simulink model "PMSM"  (R2015b)
settings: Solver=ode4  StartTime=0.0  StopTime=2  FixedStep=5e-06  RelTol=1e-5  AbsTol=1e-3
undefined symbols (not defined in the file or in its folder): DiscIntNeverNeededParam
libraries: dspmtrx3 x11, aerolibutil x7, simulink x4, simulink_extras x4, commnoisgen2 x2, dspinverses x1
(part 1 of 2)
settings Model: Creator=Сергей  LastModifiedBy=acsl
settings SolverCC: ZeroCrossAlgorithm=Adaptive
settings DataIOCC: FinalStateName=pmsm_fstate  InitialState=pmsm_fstate  LimitDataPoints=off  SaveFinalState=on  SaveCompleteFinalSimState=on  SaveFormat=Array  SignalLoggingSaveFormat=ModelDataLogs  SaveOutput=off  SignalLogging=off  DSMLogging=off  SaveTime=off  ReturnWorkspaceOutputs=on  ReturnWorkspaceOutputsName=output
settings OptimizationCC: ExpressionDepthLimit=2147483647
settings DebuggingCC: SaveWithDisabledLinksMsg=none  SaveWithParameterizedLinksMsg=none  UnderspecifiedInitializationDetection=Classic  MergeDetectMultiDrivingBlocksExec=none  SolverPrmCheckMsg=warning  Int32ToFloatConvMsg=none  FcnCallInpInsideContextMsg=EnableAllAsWarning  UnconnectedInputMsg=none  UnconnectedOutputMsg=none  UnconnectedLineMsg=none  BusObjectLabelMismatch=none  RootOutportRequireBusObject=none  ModelReferenceDataLoggingMessage=none  StateNameClashWarn=warning  SFUnusedDataAndEventsDiag=none  SFUnexpectedBacktrackingDiag=none  SFInvalidInputDataAccessInChartInitDiag=none  SFNoUnconditionalDefaultTransitionDiag=none  SFTransitionOutsideNaturalParentDiag=none  SFUnconditionalTransitionShadowingDiag=none  SFUndirectedBroadcastEventsDiag=none  SFTransitionActionBeforeConditionDiag=none
settings HardwareCC: ProdBitPerPointer=32  ProdLargestAtomicFloat=None  ProdIntDivRoundTo=Undefined  ProdEndianess=Unspecified  ProdWordSize=32  ProdHWDeviceType=32-bit Generic
settings GRTTargetCC: GeneratePreprocessorConditionals=Disable all  CombineOutputUpdateFcns=off  GRTInterface=on
settings ConfigComp: CovModelRefEnable=Off

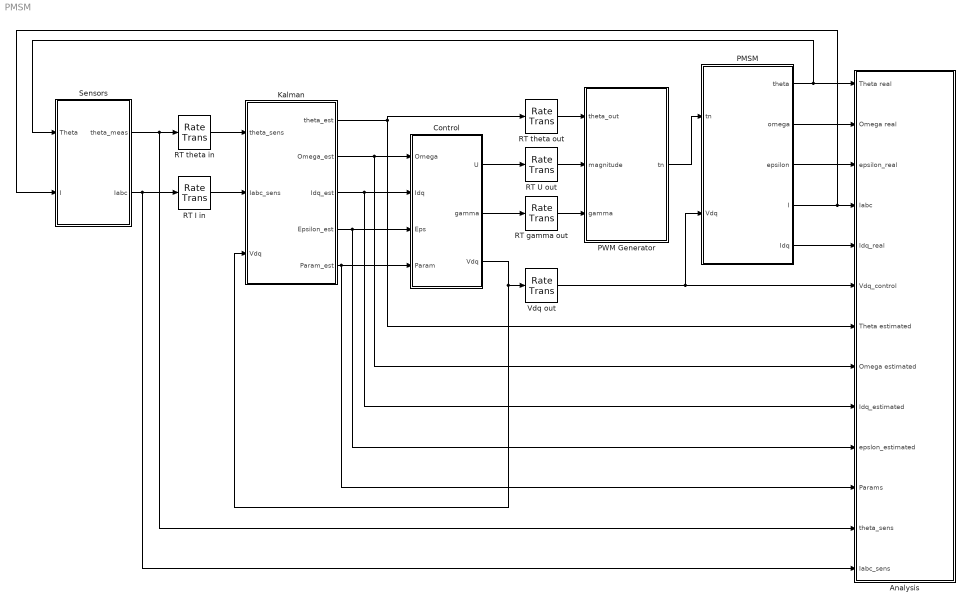
== system PMSM ==
  Analysis : Subsystem  mask{sampleTime=5e-05}
      mask prompts: sampleTime "Sample time"
  Control : Subsystem  TreatAsAtomicUnit=on  SystemSampleTime=5e-05  mask{CT=Torque control, DV=100, DT=0.06, Vs=12, R=0.4, L=0.0001, J=0.008, Kt=0.011, Kf=0.0001, Tr=2e-4, Tr_omega=1e-2, Tr_trq=3e-4, Imax=20, Wmax=110, controlST=5e-05}
      mask prompts: CT "Control type"; DV "Desired angular velocity, rev/min"; DT "Desired torque, Nm"; Vs "Nominal voltage (assumed in a model), V"; R "Coil resistance (assumed in a model), Ohm"; L "Coil inductance (assumed in a model), H"; J "Rotor inertia (assumed in a model), kg*m^2"; Kt "Torque constant (assumed in a model), N*m/A"; Kf "Viscous Friction constant (assumed in a model), N*m*s"; Tr "Rise time (velocity)"; Tr_omega "Rise time (omega)"; Tr_trq "Rise time (torque)"; Imax "I constraint"; Wmax "W constraint"; controlST "Control Sample Time"
      settings: MinAlgLoopOccurrences=on
      mask TypeOptions CT: Velocity control | Torque control
      mask Callback CT:
      | sys_name=gcs;
      | b = get_param(strcat(sys_name,'/Control'),'MaskValues');
      | a = get_param(strcat(sys_name,'/Control'),'MaskVisibilities');
      | if strcmp(b(1), 'Torque control')
      |     a{2}='off';
      |     a{3}='on';
      | end
      | if strcmp(b(1), 'Velocity control')
      |     a{2}='on';
      |     a{3}='off';
      | end
      | set_param(strcat(sys_name,'/Control'),'MaskVisibilities',a);
  Kalman : Subsystem  TreatAsAtomicUnit=on  SystemSampleTime=5e-05  mask{aaaaaa=off, Vs_r=12, Vs=12, R_r=0.3, R=0.4, L_r=0.0001, L=0.0001, J_r=0.008, J=0.008, Kt_r=0.011, Kt=0.011, Kf_r=0.001509, Kf=0.0001, Kc_r=0.010142, Kc=0.01, source=Mask, I_0=[0 0 0], I_0_r=[1 2 -3], theta0=0, theta0_r=0, w0=0, w0_r=0, eps0=0, eps0_r=0, kalmanST=5e-05}
      mask prompts: aaaaaa "Assume model parameters equal to real"; Vs_r "Nominal voltage, V"; Vs "Nominal voltage (assumed in a model), V"; R_r "Coil resistance, Ohm"; R "Coil resistance (assumed in a model), Ohm"; L_r "Coil inductance, H"; L "Coil inductance (assumed in a model), H"; J_r "Rotor inertia, kg*m^2"; J "Rotor inertia (assumed in a model), kg*m^2"; Kt_r "Torque constant, N*m/A"; Kt "Torque constant (assumed in a model), N*m/A"; Kf_r "Viscous Friction constant, N*m*s"; Kf "Viscous Friction constant (assumed in a model), N*m*s"; Kc_r "Coulomb Friction constant, N*m"; Kc "Coulomb Friction constant (assumed in a model), N*m"; source "Angle and Current initial conditions source"; I_0 "Initial currents ABC, A (assumed in a model), A"; I_0_r "Initial currents ABC, A"; theta0 "Initial angle (assumed in a model), deg"; theta0_r "Initial angle, deg"; w0 "Initial angular velocity (assumed in a model), rev/min"; w0_r "Initial angular velocity, rev/min"; eps0 "Initial angular acceleration (assumed in a model), rad/sec^2"; eps0_r "Initial angular acceleration, rad/sec^2"; kalmanST "Kalman Sample Tine"
      mask init:
      | sys_name=gcs;
      | ap = get_param(strcat(sys_name,'/PMSM'),'MaskPrompts');
      | bp = get_param(strcat(sys_name,'/Kalman'),'MaskPrompts');
      | cp = get_param(strcat(sys_name,'/Control'),'MaskPrompts');
      | a = get_param(strcat(sys_name,'/PMSM'),'MaskValues');
      | b = get_param(strcat(sys_name,'/Kalman'),'MaskValues');
      | c = get_param(strcat(sys_name,'/Control'),'MaskValues');
      | 
      | for i=1:length(ap)
      |     for j=1:length(bp)
      |         if strcmp(ap(i),bp(j))
      |             a(i)=b(j);
      |         end
      |     end
      | end
      | 
      | for i=1:length(bp)
      |     for j=1:length(cp)
      |         if strcmp(bp(i),cp(j))
      |             c(j)=b(i);
      |         end
      |     end
      | end
      | 
      | set_param(strcat(sys_name,'/PMSM'),'MaskValues',a);
      | set_param(strcat(sys_name,'/Control'),'MaskValues',c);
      settings: MinAlgLoopOccurrences=on
      mask Callback aaaaaa:
      | sys_name=gcs;
      | b = get_param(strcat(sys_name,'/Kalman'),'MaskValues');
      | 
      | if strcmp(b(1),'on')
      |     for i=3:2:19
      |         b(i)=b(i-1);
      |     end
      | end
      | 
      | set_param(strcat(sys_name,'/Kalman'),'MaskValues',b);
      mask TypeOptions source: Mask | Sensors
      mask Callback source:
      | sys_name=gcs;
      | b = get_param(strcat(sys_name,'/Kalman'),'MaskValues');
      | a = get_param(strcat(sys_name,'/Kalman'),'MaskEnables');
      | if strcmp(b(16), 'Mask')
      |     a{17}='on';
      |     a{19}='on';
      | end
      | if strcmp(b(16), 'Sensors')
      |     a{17}='off';
      |     a{19}='off';
      | end
      | set_param(strcat(sys_name,'/Kalman'),'MaskEnables',a);
  PMSM : Subsystem  mask{Vs=12, R=0.3, L=0.0001, J=0.008, Kt=0.011, Kf=0.001509, Kc=0.010142, s=0.9e-3, ws=1e-3, I_0=[1 2 -3], theta0=0, w0=0, eps0=0, delta_phin=[0 0 0]}
      mask prompts: Vs "Nominal voltage, V"; R "Coil resistance, Ohm"; L "Coil inductance, H"; J "Rotor inertia, kg*m^2"; Kt "Torque constant, N*m/A"; Kf "Viscous Friction constant, N*m*s"; Kc "Coulomb Friction constant, N*m"; s "Stribeck coeffitient, N*m"; ws "Stribeck velosity, 1/s"; I_0 "Initial currents ABC, A"; theta0 "Initial angle, deg"; w0 "Initial angular velocity, rev/min"; eps0 "Initial angular acceleration, rad/sec^2"; delta_phin "Error in phases angles, deg"
  PWM Generator : Subsystem  mask{f=40000, Vs=12}
      mask prompts: f "PWM fequency, Hz"; Vs "Nominal voltage, V"
  RT I in : RateTransition  OutPortSampleTime=5e-05
  RT U out : RateTransition  OutPortSampleTime=5e-06
  RT gamma out : RateTransition  OutPortSampleTime=5e-06
  RT theta in : RateTransition  OutPortSampleTime=5e-05
  RT theta out : RateTransition  OutPortSampleTime=5e-06
  Sensors : Subsystem  mask{I_n=[0.05 0.05 0.05], I_b=[0 0 0], D_I=0.05, h_n=[0.6 0.6 0.6]*2, h_b=[0 0 0], h_A=[3800 3800 3800], h_o=[2000 2000 2000], rrr=off, hb=[0 0 0], hA=[3800 3800 3800], ho=[2000 2000 2000], h1l=[1000 3000], h2l=[1000 3000], h3l=[1000 3000]}
      mask prompts: I_n "Coil currents fluctation error [I1 I2 I3] (3 sigma), A"; I_b "Coil currents bias [I1 I2 I3], A"; D_I "Coil currents ADC digit size, A"; h_n "Hall sensors fluctation error [H1 H2 H3] (3 sigma), ADC digits"; h_b "Hall sensors  bias [H1 H2 H3], deg"; h_A "Hall sesors ADC digits amplitude [H1 H2 H3],  ADC digits"; h_o "Hall sensors ADC digit cetral line offset [H1 H2 H3], ADC digits"; rrr "Assume etimated parameters equal to real"; hb "Hall sensors  bias [H1 H2 H3], deg"; hA "Hall sesors ADC digits amplitude [H1 H2 H3],  ADC digits"; ho "Hall sensors ADC digit cetral line offset [H1 H2 H3], ADC digits"; h1l "Hall sensor 1 trust limit"; h2l "Hall sensor 2 trust limit"; h3l "Hall sensor 3 trust limit"
      mask init:
      | ap = get_param('PMSM/Sensors','MaskPrompts');
      | a = get_param('PMSM/Sensors','MaskValues');
      | 
      | if strcmp(a(8), 'on')
      |     
      | for i=1:length(ap)
      |     for j=i:length(ap)
      |         if strcmp(ap(i),ap(j))
      |             a(j)=a(i);
      |         end
      |     end
      | end
      | 
      | end
      | 
      | set_param('PMSM/Sensors','MaskValues',a);
      mask Callback rrr:
      | sys_name=gcs;
      | ap = get_param(strcat(sys_name,'/Sensors'),'MaskPrompts');
      | a = get_param(strcat(sys_name,'/Sensors'),'MaskValues');
      | 
      | if strcmp(a(8), 'on')
      | 
      | for i=1:length(ap)
      |     for j=i:length(ap)
      |         if strcmp(ap(i),ap(j))
      |             a(j)=a(i);
      |         end
      |     end
      | end
      | 
      | end
      | 
      | set_param(strcat(sys_name,'/Sensors'),'MaskValues',a);
  Vdq out : RateTransition  OutPortSampleTime=5e-06
  wires:
  PMSM/2(omega) -> Analysis/2(Omega real)
  PMSM/3(epsilon) -> Analysis/3(epsilon_real)
  Kalman/2(Omega_est) -> Analysis/8(Omega estimated), Control/1(Omega)
  Kalman/1(theta_est) -> Analysis/7(Theta estimated), RT theta out/1
  Kalman/3(Idq_est) -> Analysis/9(Idq_estimated), Control/2(Idq)
  PMSM/5(Idq) -> Analysis/5(Idq_real)
  Kalman/4(Epsilon_est) -> Analysis/10(epslon_estimated), Control/3(Eps)
  Control/3(Vdq) -> Kalman/3(Vdq), Vdq out/1
  PWM Generator/1(tn) -> PMSM/1(tn)
  Control/2(gamma) -> RT gamma out/1
  Control/1(U) -> RT U out/1
  RT U out/1 -> PWM Generator/2(magnitude)
  RT gamma out/1 -> PWM Generator/3(gamma)
  Vdq out/1 -> PMSM/2(Vdq), Analysis/6(Vdq_control)
  PMSM/1(theta) -> Sensors/1(Theta), Analysis/1(Theta real)
  PMSM/4(I) -> Sensors/2(I), Analysis/4(Iabc)
  Sensors/1(theta_meas) -> RT theta in/1, Analysis/12(theta_sens)
  Sensors/2(Iabc) -> RT I in/1, Analysis/13(Iabc_sens)
  RT theta in/1 -> Kalman/1(theta_sens)
  RT I in/1 -> Kalman/2(Iabc_sens)
  RT theta out/1 -> PWM Generator/1(theta_out)
  Kalman/5(Param_est) -> Analysis/11(Params), Control/4(Param)

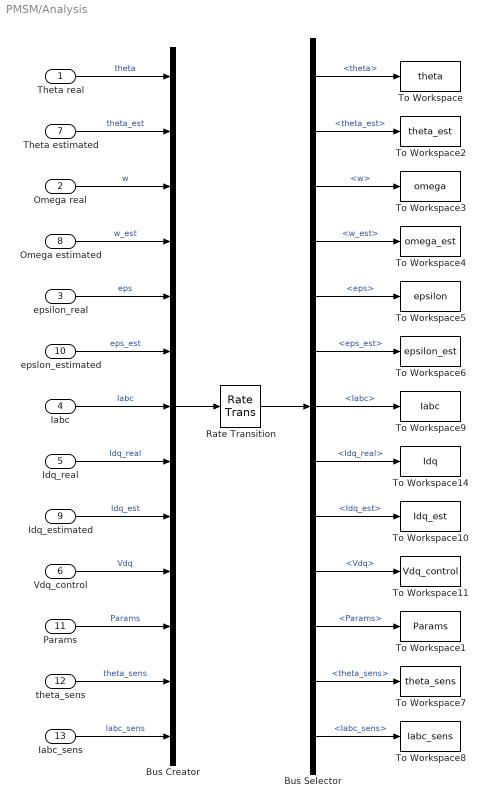
== system PMSM/Analysis ==
  Theta real : Inport
  Omega real : Inport  Port=2
  epsilon_real : Inport  Port=3
  Iabc : Inport  Port=4
  Idq_real : Inport  Port=5
  Vdq_control : Inport  Port=6
  Theta estimated : Inport  Port=7
  Omega estimated : Inport  Port=8
  Idq_estimated : Inport  Port=9
  epslon_estimated : Inport  Port=10
  Params : Inport  Port=11
  theta_sens : Inport  Port=12
  Iabc_sens : Inport  Port=13
  Bus Creator : BusCreator  Inputs=13
  Bus Selector : BusSelector  OutputSignals=theta,theta_est,w,w_est,eps,eps_est,Iabc,Idq_real,Idq_est,Vdq,Params,theta_sens,Iabc_sens
  Rate Transition : RateTransition  Deterministic=off  OutPortSampleTime=sampleTime
  To Workspace : ToWorkspace  VariableName=theta  SaveFormat=Timeseries  SampleTime=sampleTime
  To Workspace1 : ToWorkspace  VariableName=Params  SaveFormat=Timeseries  SampleTime=sampleTime
  To Workspace10 : ToWorkspace  VariableName=Idq_est  SaveFormat=Timeseries  SampleTime=sampleTime
  To Workspace11 : ToWorkspace  VariableName=Vdq_control  SaveFormat=Timeseries  SampleTime=sampleTime
  To Workspace14 : ToWorkspace  VariableName=Idq  SaveFormat=Timeseries  SampleTime=sampleTime
  To Workspace2 : ToWorkspace  VariableName=theta_est  SaveFormat=Timeseries  SampleTime=sampleTime
  To Workspace3 : ToWorkspace  VariableName=omega  SaveFormat=Timeseries  SampleTime=sampleTime
  To Workspace4 : ToWorkspace  VariableName=omega_est  SaveFormat=Timeseries  SampleTime=sampleTime
  To Workspace5 : ToWorkspace  VariableName=epsilon  SaveFormat=Timeseries  SampleTime=sampleTime
  To Workspace6 : ToWorkspace  VariableName=epsilon_est  SaveFormat=Timeseries  SampleTime=sampleTime
  To Workspace7 : ToWorkspace  VariableName=theta_sens  SaveFormat=Timeseries  SampleTime=sampleTime
  To Workspace8 : ToWorkspace  VariableName=Iabc_sens  SaveFormat=Timeseries  SampleTime=sampleTime
  To Workspace9 : ToWorkspace  VariableName=Iabc  SaveFormat=Timeseries  SampleTime=sampleTime
  wires:
  Theta estimated/1 -> Bus Creator/2  "theta_est"
  Theta real/1 -> Bus Creator/1  "theta"
  epsilon_real/1 -> Bus Creator/5  "eps"
  Iabc/1 -> Bus Creator/7  "Iabc"
  Bus Creator/1 -> Rate Transition/1
  Rate Transition/1 -> Bus Selector/1
  Bus Selector/1 -> To Workspace/1  "<theta>"
  Omega real/1 -> Bus Creator/3  "w"
  epslon_estimated/1 -> Bus Creator/6  "eps_est"
  Idq_estimated/1 -> Bus Creator/9  "Idq_est"
  Vdq_control/1 -> Bus Creator/10  "Vdq"
  Bus Selector/3 -> To Workspace3/1  "<w>"
  Bus Selector/4 -> To Workspace4/1  "<w_est>"
  Bus Selector/5 -> To Workspace5/1  "<eps>"
  Bus Selector/6 -> To Workspace6/1  "<eps_est>"
  Bus Selector/7 -> To Workspace9/1  "<Iabc>"
  Bus Selector/9 -> To Workspace10/1  "<Idq_est>"
  Bus Selector/10 -> To Workspace11/1  "<Vdq>"
  Omega estimated/1 -> Bus Creator/4  "w_est"
  Idq_real/1 -> Bus Creator/8  "Idq_real"
  Bus Selector/8 -> To Workspace14/1  "<Idq_real>"
  Bus Selector/2 -> To Workspace2/1  "<theta_est>"
  Params/1 -> Bus Creator/11  "Params"
  Bus Selector/11 -> To Workspace1/1  "<Params>"
  theta_sens/1 -> Bus Creator/12  "theta_sens"
  Iabc_sens/1 -> Bus Creator/13  "Iabc_sens"
  Bus Selector/12 -> To Workspace7/1  "<theta_sens>"
  Bus Selector/13 -> To Workspace8/1  "<Iabc_sens>"

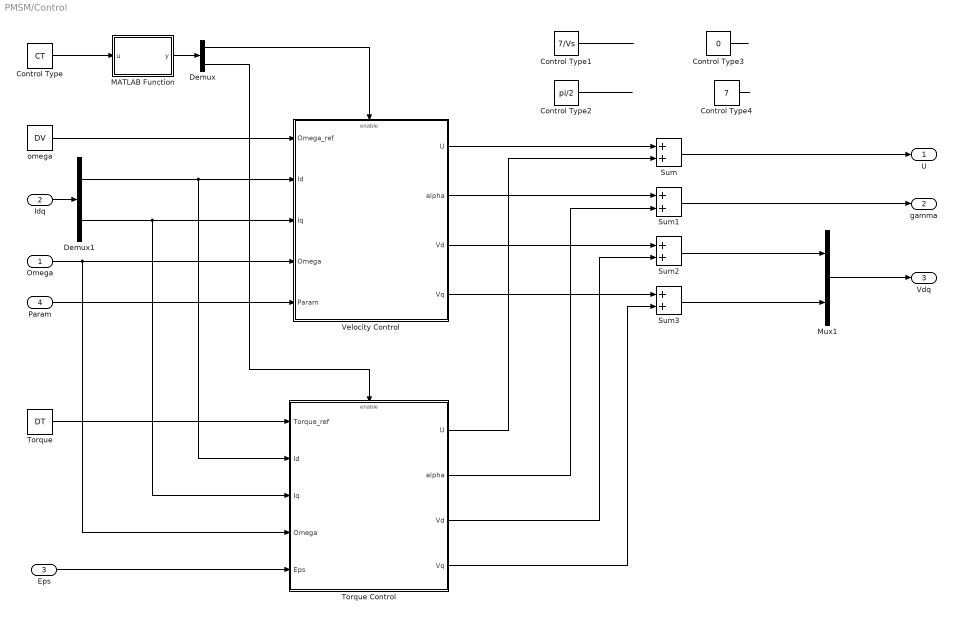
== system PMSM/Control ==
  Omega : Inport
  Idq : Inport  Port=2
  Eps : Inport  Port=3
  Param : Inport  Port=4
  Control Type : Constant  Value=CT
  Control Type1 : Constant  Value=7/Vs
  Control Type2 : Constant  Value=pi/2
  Control Type3 : Constant  Value=0
  Control Type4 : Constant  Value=7
  Demux : Demux  Outputs=2
  Demux1 : Demux  Outputs=2
  MATLAB Function : MATLAB Function  TreatAsAtomicUnit=on
  Mux1 : Mux  Inputs=2
  Sum{,1..3} (4 alike) : Sum
  Torque : Constant  Value=DT
  Torque Control : Subsystem
  Velocity Control : Subsystem
  omega : Constant  Value=DV
  U : Outport
  gamma : Outport  Port=2
  Vdq : Outport  Port=3
  wires:
  omega/1 -> Velocity Control/1(Omega_ref)
  Omega/1 -> Torque Control/4(Omega), Velocity Control/4(Omega)
  Velocity Control/1(U) -> Sum/1
  Velocity Control/2(alpha) -> Sum1/1
  Velocity Control/3(Vd) -> Sum2/1
  Velocity Control/4(Vq) -> Sum3/1
  Control Type/1 -> MATLAB Function/1(u)
  Torque/1 -> Torque Control/1(Torque_ref)
  MATLAB Function/1(y) -> Demux/1
  Demux/1 -> Velocity Control/Enable
  Torque Control/1(U) -> Sum/2
  Torque Control/2(alpha) -> Sum1/2
  Torque Control/3(Vd) -> Sum2/2
  Torque Control/4(Vq) -> Sum3/2
  Idq/1 -> Demux1/1
  Demux1/1 -> Torque Control/2(Id), Velocity Control/2(Id)
  Demux1/2 -> Torque Control/3(Iq), Velocity Control/3(Iq)
  Sum/1 -> U/1
  Sum1/1 -> gamma/1
  Sum2/1 -> Mux1/1
  Sum3/1 -> Mux1/2
  Eps/1 -> Torque Control/5(Eps)
  Control Type3/1 -> ?
  Control Type4/1 -> ?
  Demux/2 -> Torque Control/Enable
  Control Type1/1 -> ?
  Control Type2/1 -> ?
  Mux1/1 -> Vdq/1
  Param/1 -> Velocity Control/5(Param)

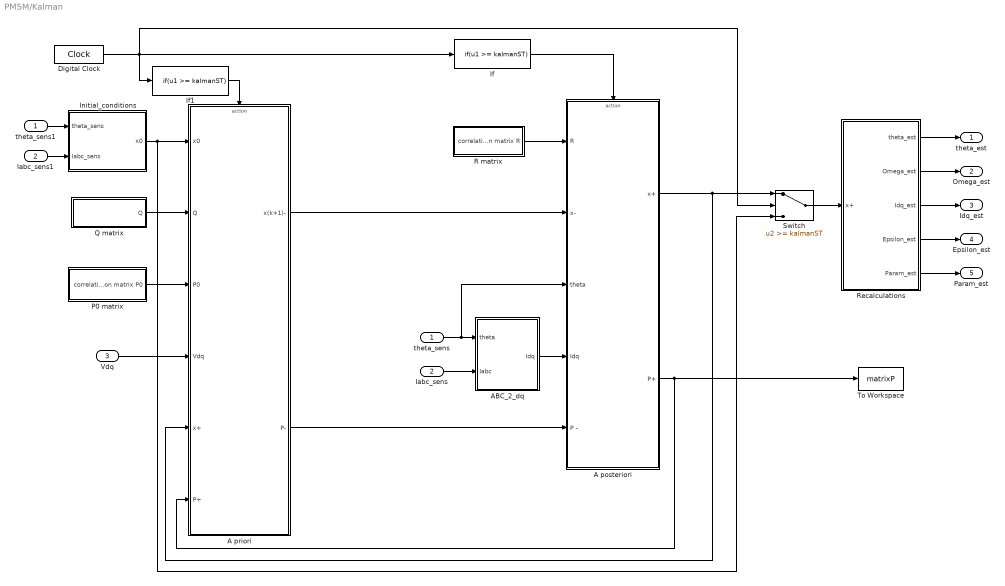
== system PMSM/Kalman ==
  theta_sens : Inport
  Iabc_sens : Inport  Port=2
  Vdq : Inport  Port=3
  A posteriori : Subsystem
  A priori : Subsystem
  ABC_2_dq : Subsystem
  Digital Clock : DigitalClock  SampleTime=kalmanST
  Iabc_sens1 : InportShadow  Port=2
  If : If  IfExpression=u1 >= kalmanST  ShowElse=off
  If1 : If  IfExpression=u1 >= kalmanST  ShowElse=off
  Initial_conditions : Subsystem
  P0 matrix : Subsystem
  Q matrix : Subsystem
  R matrix : Subsystem
  "Recalculations " : Subsystem
  Switch : Switch  Threshold=kalmanST
  To Workspace : ToWorkspace  VariableName=matrixP  SaveFormat=Timeseries  SampleTime=-1
  theta_sens1 : InportShadow
  theta_est : Outport
  Omega_est : Outport  Port=2
  Idq_est : Outport  Port=3
  Epsilon_est : Outport  Port=4
  Param_est : Outport  Port=5
  wires:
  A posteriori/1(x+) -> A priori/5(x+), Switch/1
  P0 matrix/1(correlation matrix P0) -> A priori/3(P0)
  A priori/1(x(k+1)-) -> A posteriori/2(x-)
  A posteriori/2(P+) -> To Workspace/1, A priori/6(P+)
  Q matrix/1(Q) -> A priori/2(Q)
  R matrix/1(correlation matrix R) -> A posteriori/1(R)
  A priori/2(P-) -> A posteriori/5(P -)
  theta_sens/1 -> A posteriori/3(theta), ABC_2_dq/1(theta)
  If/1 -> A posteriori/Action
  Vdq/1 -> A priori/4(Vdq)
  Digital Clock/1 -> Switch/2, If/1, If1/1
  If1/1 -> A priori/Action
  ABC_2_dq/1(Idq) -> A posteriori/4(Idq)
  Iabc_sens/1 -> ABC_2_dq/2(Iabc)
  "Recalculations "/4(Epsilon_est) -> Epsilon_est/1
  "Recalculations "/5(Param_est) -> Param_est/1
  "Recalculations "/3(Idq_est) -> Idq_est/1
  "Recalculations "/2(Omega_est) -> Omega_est/1
  "Recalculations "/1(theta_est) -> theta_est/1
  theta_sens1/1 -> Initial_conditions/1(theta_sens)
  Iabc_sens1/1 -> Initial_conditions/2(Iabc_sens)
  Switch/1 -> "Recalculations "/1(x+)
  Initial_conditions/1(x0) -> Switch/3, A priori/1(x0)

== system PMSM/PMSM ==
  tn : Inport
  Vdq : Inport  Port=2
  ABC_2_dq : Subsystem
  Degrees to Radians : simulink_extras/Transformations/Degrees to Radians
  Dot Product1 : DotProduct  InputSameDT=on  OutDataTypeStr=Inherit: Inherit via internal rule
  Kt : Gain  Gain=Kt
  Kt1 : Gain  Gain=-1
  Product : Product
  Rotor : Subsystem
  Stator : Subsystem
  Sum : Sum  Inputs=+++
  Trigonometric Function : Trigonometry
  dq_2_ABC : Subsystem
  phin : Constant  Value=[0 -2*pi/3 2*pi/3]
  phin1 : Constant  Value=delta_phin
  theta : Outport
  omega : Outport  Port=2
  epsilon : Outport  Port=3
  I : Outport  Port=4
  Idq : Outport  Port=5
  wires:
  Kt/1 -> Kt1/1, Product/1
  Rotor/3(omega) -> omega/1, Product/2
  Product/1 -> Stator/1(En)
  Trigonometric Function/1 -> Kt/1
  Sum/1 -> Trigonometric Function/1
  phin/1 -> Sum/2
  Dot Product1/1 -> Rotor/1(Te)
  Rotor/1(epsilon) -> epsilon/1
  Kt1/1 -> Dot Product1/1
  Rotor/2(theta) -> theta/1, ABC_2_dq/1(theta), dq_2_ABC/1(theta), Sum/3
  ABC_2_dq/1(Idq) -> Idq/1
  Stator/1(I) -> ABC_2_dq/2(Iabc), I/1, Dot Product1/2
  phin1/1 -> Degrees to Radians/1
  Degrees to Radians/1 -> Sum/1
  tn/1 -> Stator/2(tn)
  Vdq/1 -> dq_2_ABC/2(Vdq)
  dq_2_ABC/1(Vabc) -> Stator/3(Vabc)

== system PMSM/PWM Generator ==
  theta_out : Inport
  magnitude : Inport  Port=2
  gamma : Inport  Port=3
  Abs1 : Abs
  Constant1 : Constant  Value=0.5
  Constant2 : Constant  Value=pi/6
  ModFunction : Subsystem
  Product : Product
  Relational Operator1 : RelationalOperator  Operator=<=  OutDataTypeStr=boolean
  Sign : Signum
  Signal Generator1 : SignalGenerator  WaveForm=sawtooth  Frequency=f
  Sum1 : Sum  Inputs=|++
  Sum2 : Sum  Inputs=-+|
  Sum3 : Sum  Inputs=-+|
  Sum4 : Sum  Inputs=-+-
  phin : Constant  Value=[0 2*pi/3 4*pi/3]
  tn : Outport
  wires:
  gamma/1 -> Sum1/1
  phin/1 -> Sum4/1
  Sum2/1 -> Sign/1
  Constant1/1 -> Sum3/1, Sum2/1
  Signal Generator1/1 -> Abs1/1
  Constant2/1 -> Sum4/3
  ModFunction/1(Out1) -> Product/2
  Sum4/1 -> ModFunction/1(In1)
  Relational Operator1/1 -> Sum2/2
  Abs1/1 -> Sum3/2
  Sum3/1 -> Relational Operator1/1
  Product/1 -> Relational Operator1/2
  theta_out/1 -> Sum1/2
  magnitude/1 -> Product/1
  Sum1/1 -> Sum4/2
  Sign/1 -> tn/1

== system PMSM/Sensors ==
  Theta : Inport
  I : Inport  Port=2
  2Pi counter : Subsystem
  Demux : Demux  Outputs=3
  Gaussian Noise Generator : commnoisgen2/Gaussian Noise Generator  m=0  d=(I_n/3).^2  s=0  Ts=5e-06  frameBased=off  sampPerFrame=1  orient=off  outDataType=double
  Hall Sensor Coder : Subsystem
  Hall sensor decoder : Subsystem
  Mux : Mux  Inputs=3
  Quantizer : Quantizer  QuantizationInterval=D_I
  Sum1 : Sum  Inputs=+++
  bias currents : Constant  Value=I_b
  theta_meas : Outport
  Iabc : Outport  Port=2
  wires:
  Sum1/1 -> Quantizer/1
  Gaussian Noise Generator/1 -> Sum1/2
  Hall Sensor Coder/1(h) -> Hall sensor decoder/1(h)
  bias currents/1 -> Sum1/3
  Hall sensor decoder/1(theta_meas) -> 2Pi counter/1(Theta)
  Quantizer/1 -> Demux/1
  Demux/1 -> Mux/1
  Demux/3 -> Mux/3
  Demux/2 -> Mux/2
  I/1 -> Sum1/1
  Theta/1 -> Hall Sensor Coder/1(theta)
  2Pi counter/1(Theta_out) -> theta_meas/1
  Mux/1 -> Iabc/1

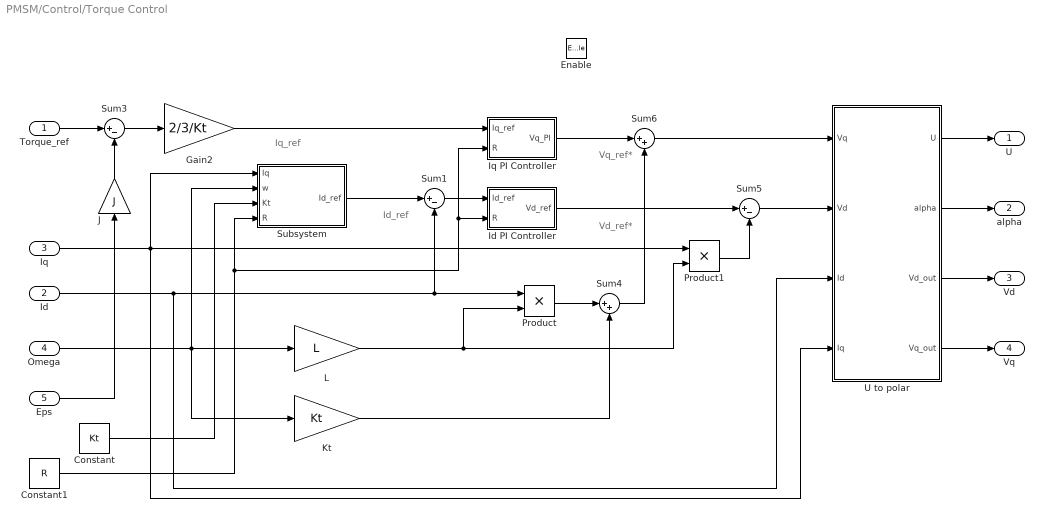
== system PMSM/Control/Torque Control ==
  note: Id_ref
  note: Iq_ref
  note: Vq_ref*
  note: Vd_ref*
  Torque_ref : Inport
  Id : Inport  Port=2
  Iq : Inport  Port=3
  Omega : Inport  Port=4
  Eps : Inport  Port=5
  Enable : EnablePort
  Constant : Constant  Value=Kt
  Constant1 : Constant  Value=R
  Gain2 : Gain  Gain=2/3/Kt
  Id PI Controller : Subsystem  mask{P=L/(Tr_trq*log(9)), I=R/(Tr_trq*log(9)), InitialConditionForIntegrator=0}
      mask prompts: P "Proportional Gain"; I "Integral Gain"; InitialConditionForIntegrator "Initial Condition For Integrator"
  Iq PI Controller : Subsystem  mask{P=L/(Tr_trq*log(9)), I=R/(Tr_trq*log(9)), InitialConditionForIntegrator=0}
      mask prompts: P "Proportional Gain"; I "Integral Gain"; InitialConditionForIntegrator "Initial Condition For Integrator"
  J : Gain  Gain=J
  Kt : Gain  Gain=Kt
  L : Gain  Gain=L
  Product : Product  RndMeth=Zero
  Product1 : Product  RndMeth=Zero
  Subsystem : Subsystem
  Sum1 : Sum  Inputs=|+-
  Sum3 : Sum  Inputs=|+-
  Sum4 : Sum  Inputs=|++
  Sum5 : Sum  Inputs=|+-
  Sum6 : Sum  Inputs=|++
  U to polar : Subsystem
  U : Outport
  alpha : Outport  Port=2
  Vd : Outport  Port=3
  Vq : Outport  Port=4
  wires:
  Sum6/1 -> U to polar/1(Vq)
  Sum3/1 -> Gain2/1
  U to polar/4(Vq_out) -> Vq/1
  U to polar/3(Vd_out) -> Vd/1
  U to polar/2(alpha) -> alpha/1
  U to polar/1(U) -> U/1
  Sum5/1 -> U to polar/2(Vd)
  Kt/1 -> Sum4/2
  Sum4/1 -> Sum6/2
  Product1/1 -> Sum5/2
  Product/1 -> Sum4/1
  L/1 -> Product/2, Product1/2
  Gain2/1 -> Iq PI Controller/1(Iq_ref)
  Sum1/1 -> Id PI Controller/1(Id_ref)
  Omega/1 -> L/1, Subsystem/2(w), Kt/1
  Torque_ref/1 -> Sum3/1
  Iq/1 -> Product1/1, Subsystem/1(Iq), U to polar/4(Iq)
  Id/1 -> Product/1, Sum1/2, U to polar/3(Id)
  Subsystem/1(Id_ref) -> Sum1/1
  Eps/1 -> J/1
  J/1 -> Sum3/2
  Constant1/1 -> Subsystem/4(R), Iq PI Controller/2(R), Id PI Controller/2(R)
  Constant/1 -> Subsystem/3(Kt)
  Iq PI Controller/1(Vq_PI) -> Sum6/1
  Id PI Controller/1(Vd_ref) -> Sum5/1

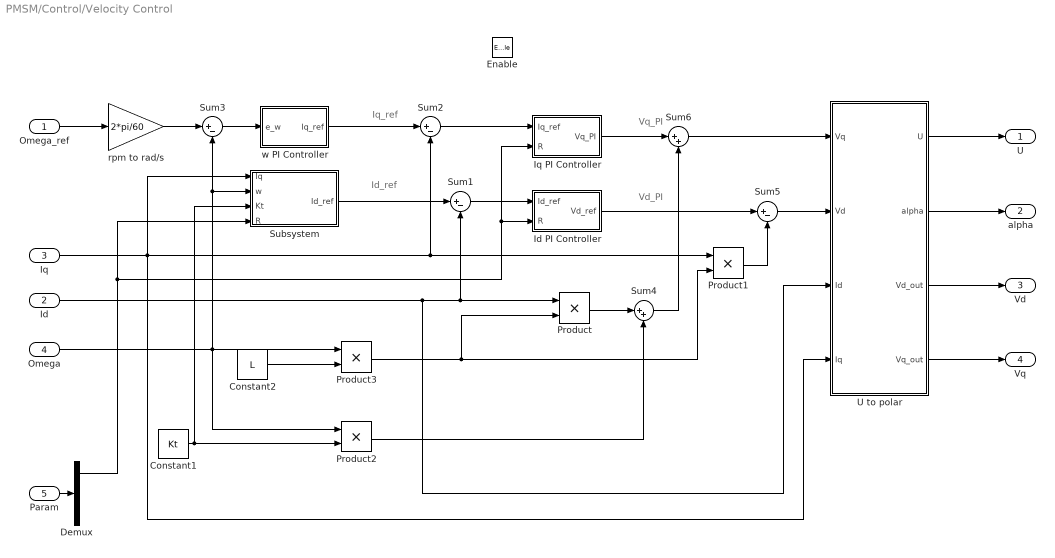
== system PMSM/Control/Velocity Control ==
  note: Id_ref
  note: Vd_PI
  note: Vq_PI
  note: Iq_ref
  Omega_ref : Inport
  Id : Inport  Port=2
  Iq : Inport  Port=3
  Omega : Inport  Port=4
  Param : Inport  Port=5
  Enable : EnablePort
  Constant1 : Constant  Value=Kt
  Constant2 : Constant  Value=L
  Demux : Demux  Outputs=3
  Id PI Controller : Subsystem  mask{P=L/(Tr*log(9)), I=R/(Tr*log(9)), InitialConditionForIntegrator=0}
      mask prompts: P "Proportional Gain"; I "Integral Gain"; InitialConditionForIntegrator "Initial Condition For Integrator"
  Iq PI Controller : Subsystem  mask{P=L/(Tr*log(9)), I=R/(Tr*log(9)), InitialConditionForIntegrator=0}
      mask prompts: P "Proportional Gain"; I "Integral Gain"; InitialConditionForIntegrator "Initial Condition For Integrator"
  Product{,1..3} (4 alike) : Product  RndMeth=Zero
  Subsystem : Subsystem
  Sum{1..3,5} (4 alike) : Sum  Inputs=|+-
  Sum4 : Sum  Inputs=|++
  Sum6 : Sum  Inputs=|++
  U to polar : Subsystem
  rpm to rad/s : Gain  Gain=2*pi/60
  w PI Controller : Subsystem  mask{P=J/(Tr_omega*log(9))^2, I=J/(Tr_omega*log(9))^2, InitialConditionForIntegrator=0}
      mask prompts: P "Proportional Gain"; I "Integral Gain"; InitialConditionForIntegrator "Initial Condition For Integrator"
  U : Outport
  alpha : Outport  Port=2
  Vd : Outport  Port=3
  Vq : Outport  Port=4
  wires:
  Subsystem/1(Id_ref) -> Sum1/1
  Sum1/1 -> Id PI Controller/1(Id_ref)
  Id/1 -> U to polar/3(Id), Product/1, Sum1/2
  Sum3/1 -> w PI Controller/1(e_w)
  Omega_ref/1 -> rpm to rad/s/1
  Omega/1 -> Product3/1, Product2/1, Sum3/2, Subsystem/2(w)
  Product3/1 -> Product1/2, Product/2
  Product/1 -> Sum4/1
  Sum4/1 -> Sum6/2
  Product2/1 -> Sum4/2
  rpm to rad/s/1 -> Sum3/1
  Product1/1 -> Sum5/2
  U to polar/1(U) -> U/1
  U to polar/2(alpha) -> alpha/1
  Sum6/1 -> U to polar/1(Vq)
  Sum5/1 -> U to polar/2(Vd)
  U to polar/3(Vd_out) -> Vd/1
  U to polar/4(Vq_out) -> Vq/1
  Sum2/1 -> Iq PI Controller/1(Iq_ref)
  Constant1/1 -> Subsystem/3(Kt), Product2/2
  Constant2/1 -> Product3/2
  Iq/1 -> Product1/1, Sum2/2, Subsystem/1(Iq), U to polar/4(Iq)
  Demux/1 -> Subsystem/4(R), Iq PI Controller/2(R), Id PI Controller/2(R)
  w PI Controller/1(Iq_ref) -> Sum2/1
  Iq PI Controller/1(Vq_PI) -> Sum6/1
  Id PI Controller/1(Vd_ref) -> Sum5/1
  Param/1 -> Demux/1

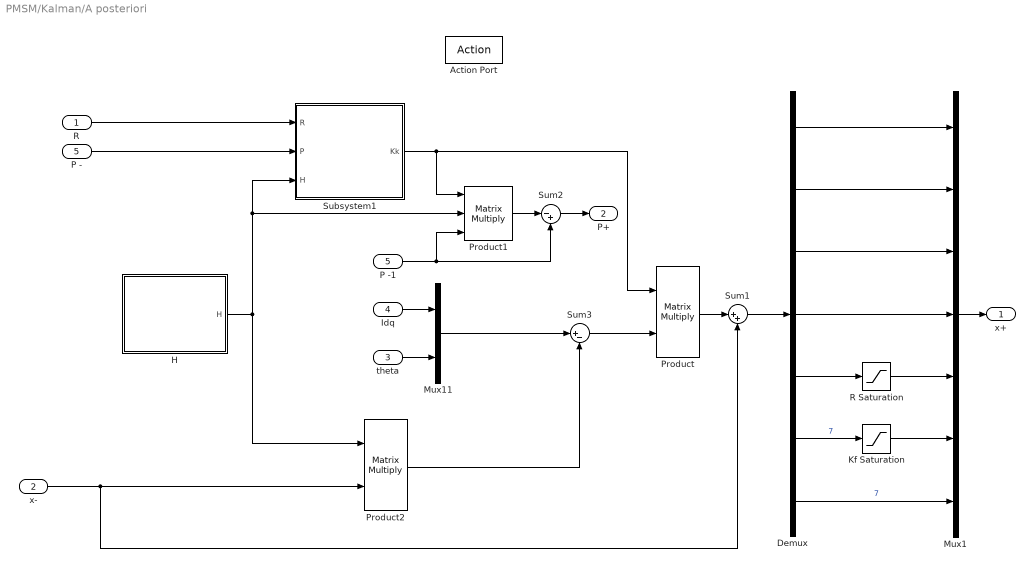
== system PMSM/Kalman/A posteriori ==
  R : Inport
  x- : Inport  Port=2
  theta : Inport  Port=3
  Idq : Inport  Port=4
  P - : Inport  Port=5
  Action Port : ActionPort  ActionType=then
  Demux : Demux  Outputs=7
  H : Subsystem
  Kf Saturation : Saturate  UpperLimit=0.1  LowerLimit=0
  Mux1 : Mux  Inputs=7
  Mux11 : Mux  Inputs=2
  P -1 : InportShadow  Port=5
  Product : Product  Multiplication=Matrix(*)  RndMeth=Zero
  Product1 : Product  Inputs=3  Multiplication=Matrix(*)  RndMeth=Zero
  Product2 : Product  Multiplication=Matrix(*)  RndMeth=Zero
  R Saturation : Saturate  UpperLimit=1  LowerLimit=0
  Subsystem1 : Subsystem
  Sum1 : Sum  Inputs=|++
  Sum2 : Sum  Inputs=|-+
  Sum3 : Sum  Inputs=|+-
  x+ : Outport
  P+ : Outport  Port=2
  wires:
  Product/1 -> Sum1/1
  P -1/1 -> Sum2/2, Product1/3
  P -/1 -> Subsystem1/2(P)
  theta/1 -> Mux11/2
  Sum3/1 -> Product/2
  Idq/1 -> Mux11/1
  Subsystem1/1(Kk) -> Product/1, Product1/1
  R/1 -> Subsystem1/1(R)
  Mux11/1 -> Sum3/1
  Product1/1 -> Sum2/1
  H/1(H) -> Product2/1, Subsystem1/3(H), Product1/2
  Sum2/1 -> P+/1
  x-/1 -> Product2/2, Sum1/2
  Mux1/1 -> x+/1
  Demux/1 -> Mux1/1
  Demux/2 -> Mux1/2
  Demux/3 -> Mux1/3
  Demux/4 -> Mux1/4
  Sum1/1 -> Demux/1
  Demux/5 -> R Saturation/1
  Product2/1 -> Sum3/2
  R Saturation/1 -> Mux1/5
  Demux/7 -> Mux1/7  "7"
  Demux/6 -> Kf Saturation/1  "7"
  Kf Saturation/1 -> Mux1/6

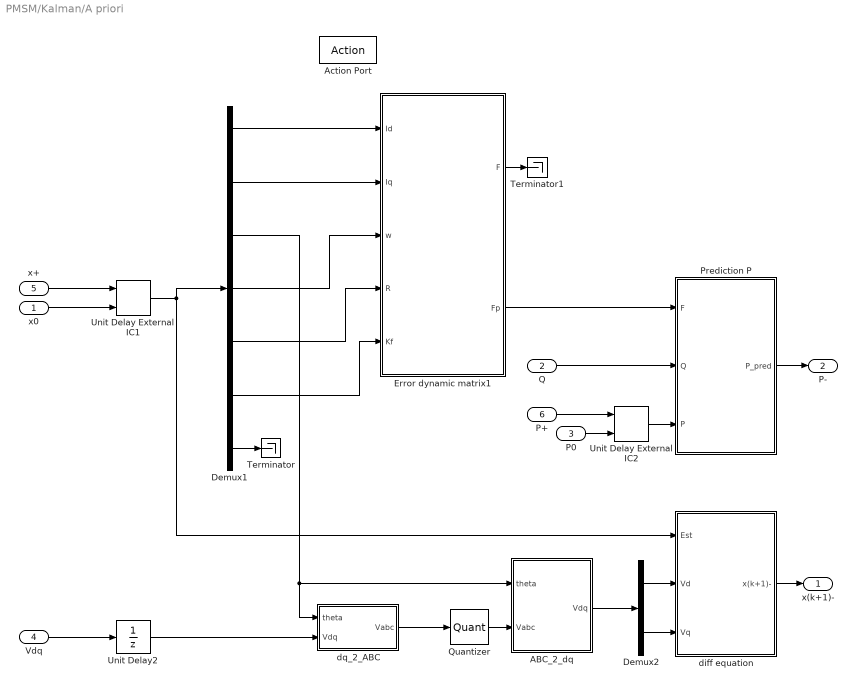
== system PMSM/Kalman/A priori ==
  x0 : Inport
  Q : Inport  Port=2
  P0 : Inport  Port=3
  Vdq : Inport  Port=4
  x+ : Inport  Port=5
  P+ : Inport  Port=6
  Action Port : ActionPort  ActionType=then
  ABC_2_dq : Subsystem
  Demux1 : Demux  Outputs=7
  Demux2 : Demux  Outputs=2
  Error dynamic matrix1 : Subsystem
  Prediction P : Subsystem
  Quantizer : Quantizer  QuantizationInterval=2*Vs*2e-8/kalmanST
  Terminator : Terminator
  Terminator1 : Terminator
  Unit Delay External IC1 : simulink/Additional Math & Discrete/Additional Discrete/Unit Delay External IC  tsamp=-1
  Unit Delay External IC2 : simulink/Additional Math & Discrete/Additional Discrete/Unit Delay External IC  tsamp=-1
  Unit Delay2 : UnitDelay  SampleTime=-1
  diff equation : Subsystem
  dq_2_ABC : Subsystem
  x(k+1)- : Outport
  P- : Outport  Port=2
  wires:
  P+/1 -> Unit Delay External IC2/1
  P0/1 -> Unit Delay External IC2/2
  Prediction P/1(P_pred) -> P-/1
  Q/1 -> Prediction P/2(Q)
  diff equation/1(x(k+1)-) -> x(k+1)-/1
  x0/1 -> Unit Delay External IC1/2
  x+/1 -> Unit Delay External IC1/1
  Vdq/1 -> Unit Delay2/1
  Unit Delay External IC2/1 -> Prediction P/3(P)
  Demux2/1 -> diff equation/2(Vd)
  Unit Delay External IC1/1 -> diff equation/1(Est), Demux1/1
  Demux2/2 -> diff equation/3(Vq)
  Demux1/1 -> Error dynamic matrix1/1(Id)
  Demux1/2 -> Error dynamic matrix1/2(Iq)
  Demux1/4 -> Error dynamic matrix1/3(w)
  ABC_2_dq/1(Vdq) -> Demux2/1
  Demux1/3 -> dq_2_ABC/1(theta), ABC_2_dq/1(theta)
  Quantizer/1 -> ABC_2_dq/2(Vabc)
  Error dynamic matrix1/2(Fp) -> Prediction P/1(F)
  Demux1/5 -> Error dynamic matrix1/4(R)
  dq_2_ABC/1(Vabc) -> Quantizer/1
  Unit Delay2/1 -> dq_2_ABC/2(Vdq)
  Demux1/6 -> Error dynamic matrix1/5(Kf)
  Demux1/7 -> Terminator/1
  Error dynamic matrix1/1(F) -> Terminator1/1

== system PMSM/Kalman/ABC_2_dq ==
  theta : Inport
  Iabc : Inport  Port=2
  Product1 : Product  Multiplication=Matrix(*)  RndMeth=Zero
  Subsystem1 : Subsystem
  Idq : Outport
  wires:
  theta/1 -> Subsystem1/1(theta)
  Subsystem1/1(A) -> Product1/1
  Product1/1 -> Idq/1
  Iabc/1 -> Product1/2

== system PMSM/Kalman/Initial_conditions ==
  theta_sens : Inport
  Iabc_sens : Inport  Port=2
  Control Type : Constant  Value=source
  Demux : Demux  Outputs=2
  Initial_conditions from mask : Subsystem
  Initial_conditions from sensors : Subsystem
  MATLAB Function : MATLAB Function  TreatAsAtomicUnit=on
  Sum : Sum
  x0 : Outport
  wires:
  Control Type/1 -> MATLAB Function/1(u)
  MATLAB Function/1(y) -> Demux/1
  Demux/1 -> Initial_conditions from mask/Enable
  Demux/2 -> Initial_conditions from sensors/Enable
  theta_sens/1 -> Initial_conditions from sensors/1(theta_sens)
  Iabc_sens/1 -> Initial_conditions from sensors/2(Iabc_sens)
  Initial_conditions from sensors/1(x0) -> Sum/2
  Initial_conditions from mask/1(x0) -> Sum/1
  Sum/1 -> x0/1

== system PMSM/Kalman/P0 matrix ==
  Create Diagonal Matrix : dspmtrx3/Create Diagonal Matrix
  Math Function : Math  Operator=square  SaturateOnIntegerOverflow=on
  Mux : Mux  Inputs=7
  sigma Id : Constant  Value=0.1
  sigma Iq : Constant  Value=0.1
  sigma Kf : Constant  Value=0.0001
  sigma R : Constant  Value=0.001
  sigma Tl : Constant  Value=0.0002
  sigma omega : Constant  Value=0.05236
  sigma theta : Constant  Value=0.0017453
  correlation matrix P0 : Outport
  wires:
  Create Diagonal Matrix/1 -> correlation matrix P0/1
  Math Function/1 -> Create Diagonal Matrix/1
  sigma omega/1 -> Mux/4
  sigma theta/1 -> Mux/3
  Mux/1 -> Math Function/1
  sigma Iq/1 -> Mux/2
  sigma Id/1 -> Mux/1
  sigma Kf/1 -> Mux/6
  sigma R/1 -> Mux/5
  sigma Tl/1 -> Mux/7

== system PMSM/Kalman/Q matrix ==
  Create Diagonal Matrix : dspmtrx3/Create Diagonal Matrix
  Math Function : Math  Operator=square  SaturateOnIntegerOverflow=on
  Mux2 : Mux  Inputs=7
  err Id : Constant  Value=0.0005
  err Iq : Constant  Value=0.0005
  err Kf : Constant  Value=1e-05
  err R : Constant  Value=1e-05
  err Tl : Constant  Value=1e-06
  err omega : Constant  Value=0.0010312
  err theta : Constant  Value=1.7453e-06
  Q : Outport
  wires:
  err omega/1 -> Mux2/4
  Math Function/1 -> Create Diagonal Matrix/1
  err theta/1 -> Mux2/3
  err Iq/1 -> Mux2/2
  err Id/1 -> Mux2/1
  err R/1 -> Mux2/5
  err Tl/1 -> Mux2/7
  Create Diagonal Matrix/1 -> Q/1
  Mux2/1 -> Math Function/1
  err Kf/1 -> Mux2/6

== system PMSM/Kalman/R matrix ==
  Create Diagonal Matrix : dspmtrx3/Create Diagonal Matrix
  Math Function : Math  Operator=square  SaturateOnIntegerOverflow=on
  Mux : Mux  Inputs=3
  sigma Id : Constant  Value=0.01
  sigma Iq : Constant  Value=0.01
  sigma theta : Constant  Value=0.00034907
  correlation matrix R : Outport
  wires:
  sigma Iq/1 -> Mux/2
  Math Function/1 -> Create Diagonal Matrix/1
  sigma theta/1 -> Mux/3
  Create Diagonal Matrix/1 -> correlation matrix R/1
  sigma Id/1 -> Mux/1
  Mux/1 -> Math Function/1

== system PMSM/Kalman/Recalculations  ==
  x+ : Inport
  Demux : Demux  Outputs=7
  Gain : Gain  Gain=1/J
  Gain2 : Gain  Gain=1.5*Kt
  Mux1 : Mux  Inputs=2
  Mux3 : Mux  Inputs=3
  Product : Product
  Sum1 : Sum  Inputs=++|
  Sum4 : Sum  Inputs=-+|
  theta_est : Outport
  Omega_est : Outport  Port=2
  Idq_est : Outport  Port=3
  Epsilon_est : Outport  Port=4
  Param_est : Outport  Port=5
  wires:
  x+/1 -> Demux/1
  Demux/1 -> Mux1/1
  Demux/4 -> Omega_est/1, Product/1
  Demux/3 -> theta_est/1
  Demux/2 -> Mux1/2, Gain2/1
  Mux1/1 -> Idq_est/1
  Gain/1 -> Epsilon_est/1
  Demux/5 -> Mux3/1
  Product/1 -> Sum4/1
  Sum1/1 -> Gain/1
  Mux3/1 -> Param_est/1
  Demux/6 -> Mux3/2, Product/2
  Sum4/1 -> Mux3/3, Sum1/2
  Gain2/1 -> Sum1/1
  Demux/7 -> Sum4/2

== system PMSM/PMSM/ABC_2_dq ==
  theta : Inport
  Iabc : Inport  Port=2
  Product1 : Product  Multiplication=Matrix(*)  RndMeth=Zero
  Subsystem1 : Subsystem
  Idq : Outport
  wires:
  theta/1 -> Subsystem1/1(theta)
  Subsystem1/1(A) -> Product1/1
  Product1/1 -> Idq/1
  Iabc/1 -> Product1/2

== system PMSM/PMSM/Rotor ==
  Te : Inport
  Friction : Subsystem
  Gain1 : Gain  Gain=1/J
  Integrator : Integrator  InitialCondition=w0*2*pi/60
  Integrator1 : Integrator  InitialCondition=theta0*pi/180
  Sum : Sum  Inputs=+++
  epsilon : Outport
  theta : Outport  Port=2
  omega : Outport  Port=3
  wires:
  Integrator1/1 -> theta/1
  Sum/1 -> Gain1/1
  Te/1 -> Sum/1
  Friction/1(Viscous friction) -> Sum/2
  Friction/2(Coulomb friction) -> Sum/3
  Gain1/1 -> Integrator/1, epsilon/1
  Integrator/1 -> Integrator1/1, omega/1, Friction/1(w)

== system PMSM/PMSM/Stator ==
  note: in
  En : Inport
  tn : Inport  Port=2
  Vabc : Inport  Port=3
  Demux1 : Demux  Outputs=3
  Gain1 : Gain  Gain=1/L
  Gain2 : Gain  Gain=R
  Integrator : Integrator  InitialCondition=I_0
  Mux1 : Mux  Inputs=3
  Phase_voltage : Subsystem
  Sum1 : Sum  Inputs=-+|
  Sum2 : Sum  Inputs=++|
  I : Outport
  wires:
  Integrator/1 -> Gain2/1, Demux1/1
  Mux1/1 -> I/1
  Demux1/1 -> Mux1/1
  Demux1/2 -> Mux1/2
  Demux1/3 -> Mux1/3
  En/1 -> Sum2/1
  Sum1/1 -> Gain1/1
  Sum2/1 -> Sum1/2
  Gain1/1 -> Integrator/1
  Gain2/1 -> Sum1/1
  tn/1 -> Phase_voltage/1(tn)
  Phase_voltage/1(en) -> ?
  Vabc/1 -> Sum2/2

== system PMSM/PMSM/dq_2_ABC ==
  theta : Inport
  Vdq : Inport  Port=2
  Product1 : Product  Multiplication=Matrix(*)  RndMeth=Zero
  Subsystem : Subsystem
  Vabc : Outport
  wires:
  theta/1 -> Subsystem/1(theta)
  Subsystem/1(A^-1) -> Product1/1
  Product1/1 -> Vabc/1
  Vdq/1 -> Product1/2

== system PMSM/PWM Generator/ModFunction ==
  note: [-0.5;0.5]
  In1 : Inport
  Gain : Gain  Gain=1/sqrt(3)
  Gain2 : Gain  Gain=1/2
  MinMax : MinMax  Function=max
  MinMax1 : MinMax
  Sum3 : Sum  Inputs=+|+
  Sum4 : Sum  Inputs=|+-
  Trigonometric Function : Trigonometry  Operator=cos
  Out1 : Outport
  wires:
  Sum4/1 -> Gain/1
  Gain2/1 -> Sum4/2
  MinMax1/1 -> Sum3/2
  MinMax/1 -> Sum3/1
  Sum3/1 -> Gain2/1
  In1/1 -> Trigonometric Function/1
  Trigonometric Function/1 -> Sum4/1, MinMax1/1, MinMax/1
  Gain/1 -> Out1/1

== system PMSM/Sensors/2Pi counter ==
  Theta : Inport
  Gain : Gain  Gain=1/2/pi
  Gain1 : Gain  Gain=2*pi
  Memory1 : Memory
  Memory2 : Memory
  Rounding Function : Rounding  Operator=round
  Sum2 : Sum  Inputs=|+-
  Sum3 : Sum  Inputs=|++
  Sum4 : Sum  Inputs=|-+
  Theta_out : Outport
  wires:
  Theta/1 -> Memory2/1, Sum4/2, Sum2/1
  Gain1/1 -> Sum4/1
  Sum3/1 -> Memory1/1, Gain1/1
  Sum2/1 -> Gain/1
  Memory1/1 -> Sum3/2
  Gain/1 -> Rounding Function/1
  Rounding Function/1 -> Sum3/1
  Memory2/1 -> Sum2/2
  Sum4/1 -> Theta_out/1

== system PMSM/Sensors/Hall Sensor Coder ==
  theta : Inport
  Degrees to Radians : simulink_extras/Transformations/Degrees to Radians
  Gaussian Noise Generator : commnoisgen2/Gaussian Noise Generator  m=0  d=(h_n/3).^2  s=0  Ts=5e-06  frameBased=off  sampPerFrame=1  orient=off  outDataType=double
  Offset ADC : Constant  Value=h_o
  Offset phases : Constant  Value=[0 2*pi/3 4*pi/3]
  Quantizer : Quantizer  QuantizationInterval=1
  Sum : Sum  Inputs=+++
  Sum1 : Sum  Inputs=+++
  Trigonometric Function : Trigonometry
  amplitude ADC : Gain  Gain=h_A./2
  bias phases : Constant  Value=h_b
  h : Outport
  wires:
  theta/1 -> Sum/1
  Offset phases/1 -> Sum/2
  bias phases/1 -> Degrees to Radians/1
  Sum/1 -> Trigonometric Function/1
  amplitude ADC/1 -> Sum1/1
  Offset ADC/1 -> Sum1/2
  Sum1/1 -> Quantizer/1
  Quantizer/1 -> h/1
  Gaussian Noise Generator/1 -> Sum1/3
  Trigonometric Function/1 -> amplitude ADC/1
  Degrees to Radians/1 -> Sum/3

== system PMSM/Sensors/Hall sensor decoder ==
  h : Inport
  Amplitude  ADC : Constant  Value=hA./2
  Degrees to Radians : simulink_extras/Transformations/Degrees to Radians
  Hall cutter : Constant  Value=[h1l h2l h3l]
  MATLAB Function : MATLAB Function  TreatAsAtomicUnit=on
  bias phases : Constant  Value=hb
  offset ADC : Constant  Value=ho
  theta_meas : Outport
  wires:
  h/1 -> MATLAB Function/1(hall)
  bias phases/1 -> Degrees to Radians/1
  offset ADC/1 -> MATLAB Function/3(offset_ADC)
  Amplitude  ADC/1 -> MATLAB Function/4(amplitude_ADC)
  MATLAB Function/1(theta_meas) -> theta_meas/1
  Hall cutter/1 -> MATLAB Function/5(hall_cutter)
  Degrees to Radians/1 -> MATLAB Function/2(bias)

== system PMSM/Control/Torque Control/Id PI Controller ==
  Id_ref : Inport
  R : Inport  Port=2
  Clamping circuit : Subsystem
  Constant : Constant  DisableCoverage=on  Value=0  OutDataTypeStr=Inherit: Inherit via back propagation  PreserveConstantTs=on
  Integral Gain1 : Gain  DisableCoverage=on  Gain=1/(Tr_trq*log(9))  ParamDataTypeStr=Inherit: Inherit from 'Gain'  OutDataTypeStr=Inherit: Inherit via back propagation
  Integrator : DiscreteIntegrator  InitialCondition=InitialConditionForIntegrator  InitialConditionSetting=State (most efficient)  SampleTime=-1  OutDataTypeStr=Inherit: Inherit via back propagation  ICPrevOutput=DiscIntNeverNeededParam  ICPrevScaledInput=DiscIntNeverNeededParam
  Product : Product
  Proportional Gain : Gain  Gain=P  ParamDataTypeStr=Inherit: Inherit from 'Gain'  OutDataTypeStr=Inherit: Inherit via back propagation
  Saturation : Saturate  UpperLimit=Vs  LowerLimit=-Vs  LinearizeAsGain=off  OutMin=-Vs  OutMax=Vs
  Sum : Sum  Inputs=++|  OutDataTypeStr=Inherit: Same as first input
  Switch : Switch  Criteria=u2 > Threshold  InputSameDT=on
  Vd_ref : Outport  InitialOutput=0
  wires:
  Product/1 -> Switch/3, Clamping circuit/2(preIntegrator)
  Proportional Gain/1 -> Sum/1
  Saturation/1 -> Vd_ref/1
  Sum/1 -> Clamping circuit/1(preSat), Saturation/1
  Constant/1 -> Switch/1
  Clamping circuit/1(Clamp) -> Switch/2
  Switch/1 -> Integrator/1
  Id_ref/1 -> Product/1, Proportional Gain/1
  R/1 -> Integral Gain1/1
  Integral Gain1/1 -> Product/2
  Integrator/1 -> Sum/2

== system PMSM/Control/Torque Control/Iq PI Controller ==
  Iq_ref : Inport
  R : Inport  Port=2
  Clamping circuit : Subsystem
  Constant : Constant  DisableCoverage=on  Value=0  OutDataTypeStr=Inherit: Inherit via back propagation  PreserveConstantTs=on
  Integral Gain : Gain  DisableCoverage=on  Gain=I  ParamDataTypeStr=Inherit: Inherit from 'Gain'  OutDataTypeStr=Inherit: Inherit via back propagation
  Integral Gain1 : Gain  DisableCoverage=on  Gain=1/(Tr_trq*log(9))  ParamDataTypeStr=Inherit: Inherit from 'Gain'  OutDataTypeStr=Inherit: Inherit via back propagation
  Integrator : DiscreteIntegrator  InitialCondition=InitialConditionForIntegrator  InitialConditionSetting=State (most efficient)  SampleTime=-1  OutDataTypeStr=Inherit: Inherit via back propagation  ICPrevOutput=DiscIntNeverNeededParam  ICPrevScaledInput=DiscIntNeverNeededParam
  Product : Product
  Proportional Gain : Gain  Gain=P  ParamDataTypeStr=Inherit: Inherit from 'Gain'  OutDataTypeStr=Inherit: Inherit via back propagation
  Saturation : Saturate  UpperLimit=Vs  LowerLimit=-Vs  LinearizeAsGain=off  OutMin=-Vs  OutMax=Vs
  Sum : Sum  Inputs=++|  OutDataTypeStr=Inherit: Same as first input
  Switch : Switch  Criteria=u2 > Threshold  InputSameDT=on
  Vq_PI : Outport  InitialOutput=0
  wires:
  Switch/1 -> Integrator/1
  Clamping circuit/1(Clamp) -> Switch/2
  Constant/1 -> Switch/1
  Sum/1 -> Saturation/1, Clamping circuit/1(preSat)
  Saturation/1 -> Vq_PI/1
  Proportional Gain/1 -> Sum/1
  Integrator/1 -> Sum/2
  Product/1 -> Clamping circuit/2(preIntegrator), Switch/3
  Iq_ref/1 -> Product/1, Proportional Gain/1
  R/1 -> Integral Gain1/1
  Integral Gain1/1 -> Product/2

== system PMSM/Control/Torque Control/Subsystem ==
  Iq : Inport
  w : Inport  Port=2
  Kt : Inport  Port=3
  R : Inport  Port=4
  Constant : Constant  Value=0
  Divide : Product  Inputs=*/
  Gain : Gain  Gain=-1
  Math Function : Math  Operator=square  SaturateOnIntegerOverflow=on
  MinMax : MinMax  Function=max  Inputs=2
  Product : Product  Inputs=3
  Sqrt : Sqrt  SaturateOnIntegerOverflow=on
  Sum : Sum  Inputs=--|
  Id_ref : Outport
  wires:
  Iq/1 -> Math Function/1, Product/1
  w/1 -> Product/2
  Kt/1 -> Product/3
  R/1 -> Divide/2
  Product/1 -> Divide/1
  Divide/1 -> Sum/2
  Math Function/1 -> Sum/1
  Sum/1 -> MinMax/1
  Constant/1 -> MinMax/2
  MinMax/1 -> Sqrt/1
  Gain/1 -> Id_ref/1
  Sqrt/1 -> Gain/1

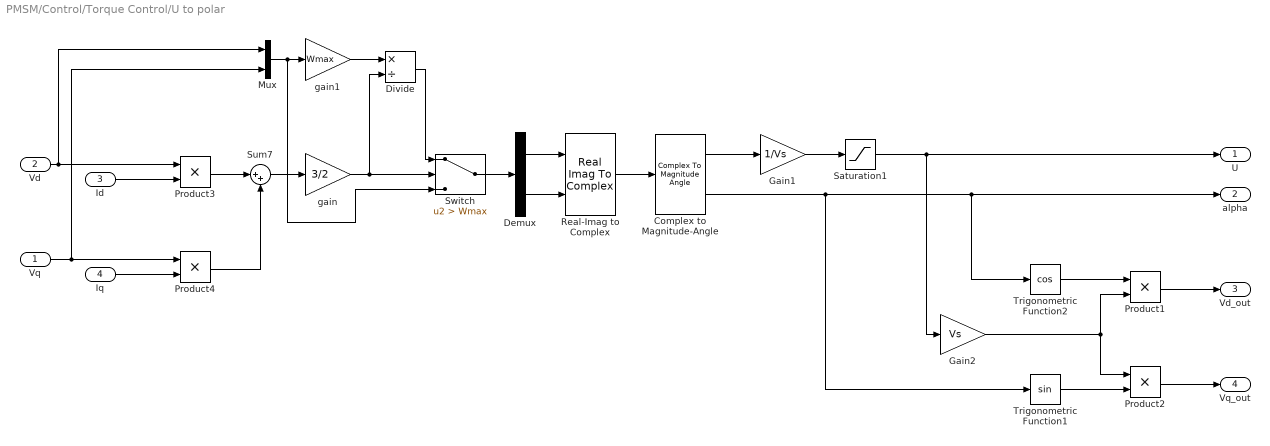
== system PMSM/Control/Torque Control/U to polar ==
  Vq : Inport
  Vd : Inport  Port=2
  Id : Inport  Port=3
  Iq : Inport  Port=4
  Complex to Magnitude-Angle : ComplexToMagnitudeAngle
  Demux : Demux  Outputs=2
  Divide : Product  Inputs=*/
  Gain1 : Gain  Gain=1/Vs
  Gain2 : Gain  Gain=Vs
  Mux : Mux  Inputs=2
  Product{1..4} (4 alike) : Product  RndMeth=Zero
  Real-Imag to Complex : RealImagToComplex
  Saturation1 : Saturate  UpperLimit=1  LowerLimit=-1
  Sum7 : Sum  Inputs=|++
  Switch : Switch  Criteria=u2 > Threshold  Threshold=Wmax
  Trigonometric Function1 : Trigonometry
  Trigonometric Function2 : Trigonometry  Operator=cos
  gain : Gain  Gain=3/2
  gain1 : Gain  Gain=Wmax
  U : Outport
  alpha : Outport  Port=2
  Vd_out : Outport  Port=3
  Vq_out : Outport  Port=4
  wires:
  Divide/1 -> Switch/1
  gain1/1 -> Divide/1
  Mux/1 -> Switch/3, gain1/1
  Demux/2 -> Real-Imag to Complex/2
  Demux/1 -> Real-Imag to Complex/1
  Switch/1 -> Demux/1
  gain/1 -> Switch/2, Divide/2
  Product3/1 -> Sum7/1
  Sum7/1 -> gain/1
  Product4/1 -> Sum7/2
  Vd/1 -> Mux/1, Product3/1
  Iq/1 -> Product4/2
  Id/1 -> Product3/2
  Product2/1 -> Vq_out/1
  Trigonometric Function1/1 -> Product2/2
  Gain2/1 -> Product1/2, Product2/1
  Product1/1 -> Vd_out/1
  Trigonometric Function2/1 -> Product1/1
  Gain1/1 -> Saturation1/1
  Saturation1/1 -> U/1, Gain2/1
  Complex to Magnitude-Angle/1 -> Gain1/1
  Vq/1 -> Product4/1, Mux/2
  Complex to Magnitude-Angle/2 -> Trigonometric Function1/1, Trigonometric Function2/1, alpha/1
  Real-Imag to Complex/1 -> Complex to Magnitude-Angle/1

== system PMSM/Control/Velocity Control/Id PI Controller ==
  Id_ref : Inport
  R : Inport  Port=2
  Clamping circuit : Subsystem
  Constant : Constant  DisableCoverage=on  Value=0  OutDataTypeStr=Inherit: Inherit via back propagation  PreserveConstantTs=on
  Integral Gain1 : Gain  DisableCoverage=on  Gain=1/(Tr*log(9))  ParamDataTypeStr=Inherit: Inherit from 'Gain'  OutDataTypeStr=Inherit: Inherit via back propagation
  Integrator : DiscreteIntegrator  InitialCondition=InitialConditionForIntegrator  InitialConditionSetting=State (most efficient)  SampleTime=-1  OutDataTypeStr=Inherit: Inherit via back propagation  ICPrevOutput=DiscIntNeverNeededParam  ICPrevScaledInput=DiscIntNeverNeededParam
  Product : Product
  Proportional Gain : Gain  Gain=P  ParamDataTypeStr=Inherit: Inherit from 'Gain'  OutDataTypeStr=Inherit: Inherit via back propagation
  Saturation : Saturate  UpperLimit=Vs  LowerLimit=-Vs  LinearizeAsGain=off  OutMin=-Vs  OutMax=Vs
  Sum : Sum  Inputs=++|  OutDataTypeStr=Inherit: Same as first input
  Switch : Switch  Criteria=u2 > Threshold  InputSameDT=on
  Vd_ref : Outport  InitialOutput=0
  wires:
  Product/1 -> Switch/3, Clamping circuit/2(preIntegrator)
  Proportional Gain/1 -> Sum/1
  Saturation/1 -> Vd_ref/1
  Sum/1 -> Clamping circuit/1(preSat), Saturation/1
  Constant/1 -> Switch/1
  Clamping circuit/1(Clamp) -> Switch/2
  Switch/1 -> Integrator/1
  Id_ref/1 -> Product/1, Proportional Gain/1
  R/1 -> Integral Gain1/1
  Integral Gain1/1 -> Product/2
  Integrator/1 -> Sum/2

== system PMSM/Control/Velocity Control/Iq PI Controller ==
  Iq_ref : Inport
  R : Inport  Port=2
  Clamping circuit : Subsystem
  Constant : Constant  DisableCoverage=on  Value=0  OutDataTypeStr=Inherit: Inherit via back propagation  PreserveConstantTs=on
  Integral Gain : Gain  DisableCoverage=on  Gain=I  ParamDataTypeStr=Inherit: Inherit from 'Gain'  OutDataTypeStr=Inherit: Inherit via back propagation
  Integral Gain1 : Gain  DisableCoverage=on  Gain=1/(Tr*log(9))  ParamDataTypeStr=Inherit: Inherit from 'Gain'  OutDataTypeStr=Inherit: Inherit via back propagation
  Integrator2 : DiscreteIntegrator  InitialCondition=InitialConditionForIntegrator  InitialConditionSetting=State (most efficient)  SampleTime=-1  OutDataTypeStr=Inherit: Inherit via back propagation  ICPrevOutput=DiscIntNeverNeededParam  ICPrevScaledInput=DiscIntNeverNeededParam
  Product : Product
  Proportional Gain : Gain  Gain=P  ParamDataTypeStr=Inherit: Inherit from 'Gain'  OutDataTypeStr=Inherit: Inherit via back propagation
  Saturation : Saturate  UpperLimit=Vs  LowerLimit=-Vs  LinearizeAsGain=off  OutMin=-Vs  OutMax=Vs
  Sum : Sum  Inputs=++|  OutDataTypeStr=Inherit: Same as first input
  Switch : Switch  Criteria=u2 > Threshold  InputSameDT=on
  Vq_PI : Outport  InitialOutput=0
  wires:
  Switch/1 -> Integrator2/1
  Clamping circuit/1(Clamp) -> Switch/2
  Constant/1 -> Switch/1
  Sum/1 -> Saturation/1, Clamping circuit/1(preSat)
  Saturation/1 -> Vq_PI/1
  Proportional Gain/1 -> Sum/1
  Product/1 -> Clamping circuit/2(preIntegrator), Switch/3
  Iq_ref/1 -> Product/1, Proportional Gain/1
  R/1 -> Integral Gain1/1
  Integral Gain1/1 -> Product/2
  Integrator2/1 -> Sum/2

== system PMSM/Control/Velocity Control/Subsystem ==
  Iq : Inport
  w : Inport  Port=2
  Kt : Inport  Port=3
  R : Inport  Port=4
  Constant : Constant  Value=0
  Constant1 : Constant  Value=4*(6e-6*Wmax/R)^2
  Divide : Product  Inputs=*/
  Gain1 : Gain  Gain=0.5
  Math Function : Math  Operator=square  SaturateOnIntegerOverflow=on
  Math Function1 : Math  Operator=square  SaturateOnIntegerOverflow=on
  MinMax : MinMax  Function=max  Inputs=2
  Mux : Mux  Inputs=2
  Product : Product  Inputs=3
  Sqrt : Sqrt  SaturateOnIntegerOverflow=on
  Sqrt1 : Sqrt  SaturateOnIntegerOverflow=on
  Sqrt2 : Sqrt  SaturateOnIntegerOverflow=on
  Sum : Sum  Inputs=--|
  Sum1 : Sum  Inputs=|++
  Sum2 : Sum  Inputs=|++
  Id_ref : Outport
  wires:
  Iq/1 -> Math Function/1, Product/1
  w/1 -> Product/2
  Kt/1 -> Product/3
  R/1 -> Divide/2
  Product/1 -> Divide/1
  Divide/1 -> Sum/2
  Math Function/1 -> Sum/1
  Sum/1 -> Sum1/1, Math Function1/1
  Math Function1/1 -> Sum2/1
  Constant1/1 -> Sum2/2
  Sum2/1 -> Sqrt1/1
  Sqrt1/1 -> Sum1/2
  Sum1/1 -> Gain1/1
  Gain1/1 -> Sqrt2/1
  Sqrt2/1 -> Id_ref/1
  ? -> MinMax/1
  Constant/1 -> MinMax/2
  MinMax/1 -> Sqrt/1
  ? -> Mux/2
  Sqrt/1 -> Mux/1

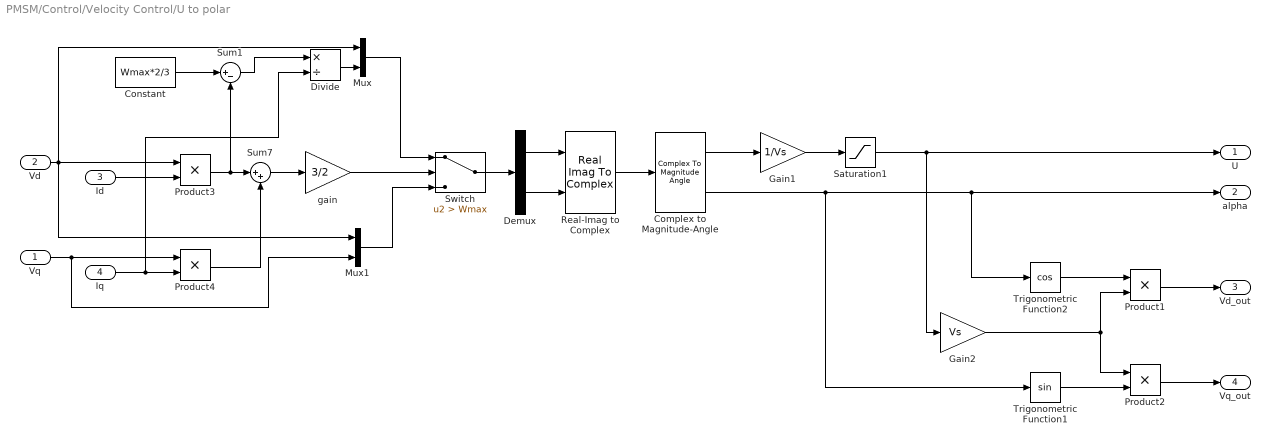
== system PMSM/Control/Velocity Control/U to polar ==
  Vq : Inport
  Vd : Inport  Port=2
  Id : Inport  Port=3
  Iq : Inport  Port=4
  Complex to Magnitude-Angle : ComplexToMagnitudeAngle
  Constant : Constant  Value=Wmax*2/3
  Demux : Demux  Outputs=2
  Divide : Product  Inputs=*/
  Gain1 : Gain  Gain=1/Vs
  Gain2 : Gain  Gain=Vs
  Mux : Mux  Inputs=2
  Mux1 : Mux  Inputs=2
  Product{1..4} (4 alike) : Product  RndMeth=Zero
  Real-Imag to Complex : RealImagToComplex
  Saturation1 : Saturate  UpperLimit=1  LowerLimit=-1
  Sum1 : Sum  Inputs=|+-
  Sum7 : Sum  Inputs=|++
  Switch : Switch  Criteria=u2 > Threshold  Threshold=Wmax
  Trigonometric Function1 : Trigonometry
  Trigonometric Function2 : Trigonometry  Operator=cos
  gain : Gain  Gain=3/2
  U : Outport
  alpha : Outport  Port=2
  Vd_out : Outport  Port=3
  Vq_out : Outport  Port=4
  wires:
  Real-Imag to Complex/1 -> Complex to Magnitude-Angle/1
  Complex to Magnitude-Angle/2 -> alpha/1, Trigonometric Function2/1, Trigonometric Function1/1
  Vq/1 -> Mux1/2, Product4/1
  Complex to Magnitude-Angle/1 -> Gain1/1
  Saturation1/1 -> Gain2/1, U/1
  Gain1/1 -> Saturation1/1
  Trigonometric Function2/1 -> Product1/1
  Product1/1 -> Vd_out/1
  Gain2/1 -> Product2/1, Product1/2
  Trigonometric Function1/1 -> Product2/2
  Product2/1 -> Vq_out/1
  Id/1 -> Product3/2
  Iq/1 -> Divide/2, Product4/2
  Vd/1 -> Mux1/1, Product3/1, Mux/1
  Product4/1 -> Sum7/2
  Sum7/1 -> gain/1
  Product3/1 -> Sum7/1, Sum1/2
  gain/1 -> Switch/2
  Switch/1 -> Demux/1
  Demux/1 -> Real-Imag to Complex/1
  Demux/2 -> Real-Imag to Complex/2
  Divide/1 -> Mux/2
  Mux1/1 -> Switch/3
  Mux/1 -> Switch/1
  Sum1/1 -> Divide/1
  Constant/1 -> Sum1/1

== system PMSM/Control/Velocity Control/w PI Controller ==
  e_w : Inport
  Clamping circuit : Subsystem
  Constant : Constant  DisableCoverage=on  Value=0  OutDataTypeStr=Inherit: Inherit via back propagation  PreserveConstantTs=on
  Demux : Demux  Outputs=2
  I limits : Subsystem
  Integral Gain : Gain  DisableCoverage=on  Gain=I  ParamDataTypeStr=Inherit: Inherit from 'Gain'  OutDataTypeStr=Inherit: Inherit via back propagation
  Integrator : DiscreteIntegrator  InitialCondition=InitialConditionForIntegrator  InitialConditionSetting=State (most efficient)  SampleTime=-1  OutDataTypeStr=Inherit: Inherit via back propagation  ICPrevOutput=DiscIntNeverNeededParam  ICPrevScaledInput=DiscIntNeverNeededParam
  Proportional Gain : Gain  Gain=P  ParamDataTypeStr=Inherit: Inherit from 'Gain'  OutDataTypeStr=Inherit: Inherit via back propagation
  Saturation Dynamic : simulink/Discontinuities/Saturation Dynamic  OutMin=[]  OutMax=[]  OutDataTypeStr=Inherit: Same as second input  OutDataType=fixdt(1, 16)  OutScaling=2^-10  DoSatur=off
  Sum : Sum  Inputs=++|  OutDataTypeStr=Inherit: Same as first input
  Switch : Switch  Criteria=u2 > Threshold  InputSameDT=on
  Iq_ref : Outport  InitialOutput=0
  wires:
  Integral Gain/1 -> Switch/3, Clamping circuit/2(preIntegrator)
  Proportional Gain/1 -> Sum/1
  Sum/1 -> Saturation Dynamic/2, Clamping circuit/1(preSat)
  Constant/1 -> Switch/1
  Clamping circuit/1(Clamp) -> Switch/2
  Switch/1 -> Integrator/1
  e_w/1 -> Integral Gain/1, Proportional Gain/1
  Saturation Dynamic/1 -> Iq_ref/1
  I limits/1(Ilimits) -> Clamping circuit/3(Ilimits), Demux/1
  Demux/1 -> Saturation Dynamic/1
  Demux/2 -> Saturation Dynamic/3
  Integrator/1 -> Sum/2

== system PMSM/Kalman/A posteriori/H ==
  " 24" : Constant  Value="[1 0 0 0 0 0 0; 0 1 0 0  0 0 0; 0 0 1 0 0 0 0]"
  H : Outport
  wires:
  " 24"/1 -> H/1
